simulink library "Single_Track_Model_linear"  (R2018b)
settings: Solver=VariableStepAuto  StartTime=0.0  StopTime=10.0  RelTol=1e-3
undefined symbols (not defined in the file): DiscIntNeverNeededParam, par_TIR, par_VEH, psi0, psip0, v0
libraries: simulink x2, vehicle_model x1
(part 1 of 2)
settings Model: Creator=Johannes  LastModifiedBy=Tony
settings SFSimCC: SimUseLocalCustomCode=off
settings RTWCC: RTWUseLocalCustomCode=off

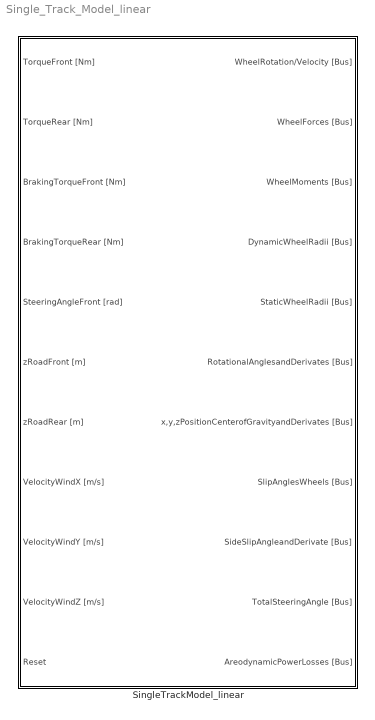
== system Single_Track_Model_linear ==
  SingleTrackModel_linear : Subsystem  mask(SB){RohAir=1.204, VEH_m=2.16e+03, VEH_Iz=5100, VEH_xSP=1.43, VEH_g=9.81, VEH_cz=0, VEH_cx=0.29, VEH_cy=0, VEH_Afront=2.24, VEH_xDP=1.43, VEH_yDP=0, VEH_l=2.968, INIT_x=0, INIT_y=0, INIT_psi=psi0, psip0=psip0, INIT_zroad_RF0=0, INIT_zroad_LF0=0, INIT_zroad_RR0=0, INIT_zroad_LR0=0, v0=v0, unloadedRadius_F=0.339750, c_alpha_F=1.034891575000098e+05, unloadedRadius_R=0.336500, c_alpha_R=1.056481395191441e+05}
      mask prompts: RohAir "Air Density [kg/m^3]"; VEH_m "Mass Vehicle [kg]"; VEH_Iz "Inertia of Vehicle about z [kg m^2]"; VEH_xSP "Center of Gravity of Vehicle in x [m]"; VEH_g "Gravity [N/kg]"; VEH_cz "cw-Value in z [-]"; VEH_cx "cw-Value in x [-]"; VEH_cy "cw-Value in y [-]"; VEH_Afront "Front Surface area [m^2]"; VEH_xDP "Pressure point position in x-direction [m]"; VEH_yDP "Pressure point position in y-direction [m]"; VEH_l "Wheel Base [m]"; INIT_x "Initial Position x"; INIT_y "Initial Position y"; INIT_psi "Initial Position psi"; psip0 "Initial psip"; INIT_zroad_RF0 "Initial Road Position z Right Front"; INIT_zroad_LF0 "Initial Road Position z Left Front"; INIT_zroad_RR0 "Initial Road Position z Right Rear"; INIT_zroad_LR0 "Initial Road Position z Left Rear"; v0 "Initial Speed [m/s]"; unloadedRadius_F "Unloaded Radius Front Tire"; c_alpha_F "Lateral Stiffness Front"; unloadedRadius_R "Unloaded Radius Rear Tire"; c_alpha_R "Lateral Stiffness Rear"
      mask help:
      | <Author> Johannes Rühm
      | <Date> 05/12/2018
      |
      | <Description>
      | Single Track Model using a linear tire model. Structure is based on double track model of "Schultze". Lateral Stiffnesses of tires must be calculated with double track model.
      |
      | <Parameters>
      | ...
      |
      | <Inputs>
      | TorqueFront [Nm]
      | TorqueRear [Nm]
      | BrakingTorqueFront [Nm]
      | BrakingTorqueRear [Nm]
      | SteeringAngleFront [rad]
      | zRoadFront [m]
      | zRoadRear [m]
      | VelocityWindX [m/s]
      | VelocityWindY [m/s]
      | VelocityWindZ [m/s]
      | Reset
      |
      | <Outputs>
      | WheelRotation/Velocity [Bus]
      | WheelForces [Bus]
      | WheelMoments [Bus]
      | DynamicWheelRadii [Bus]
      | StaticWheelRadii [Bus]
      | RotaionalAnglesandDerivatives [Bus]
      | x,y,zPositionCenterofGravityandDerivates [Bus]
      | SlipAnglesWheels [Bus]
      | SideSlipAngleandDerivate [Bus]
      | TotalSteeringAngle [Bus]
      | AreodynamicPowerLosses [Bus]
      mask init:
      | %savedec=0;
      | [par_VEH, par_TIR] =  Init_ESM_linear (RohAir,VEH_m,VEH_xSP,VEH_g,VEH_cz,VEH_cx,VEH_cy,VEH_xDP,VEH_yDP,VEH_Iz,VEH_l,VEH_Afront, unloadedRadius_F, c_alpha_F, unloadedRadius_R, c_alpha_R)
      mask DialogControl Container12 Prompt: Vehicle
      mask DialogControl Container13 Prompt: Mass Data
      mask DialogControl Container15 Prompt: Aerodynamics
      mask DialogControl Container18 Prompt: Dimensions
      mask DialogControl Container32 Prompt: Initial Parameters
      mask DialogControl Container4 Prompt: Tire
      mask DialogControl Container6 Prompt: Front
      mask DialogControl Container8 Prompt: Rear

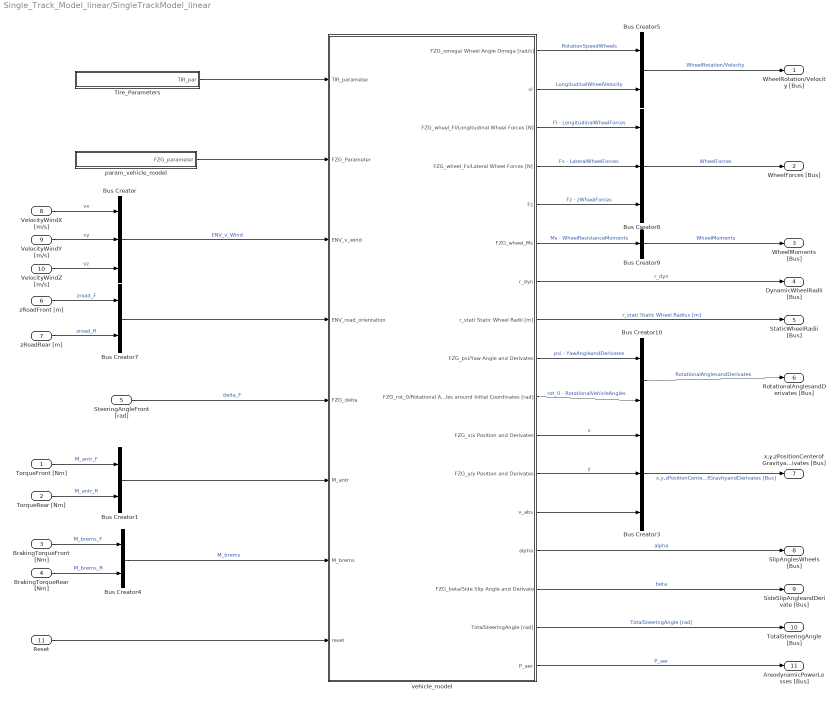
== system Single_Track_Model_linear/SingleTrackModel_linear ==
  TorqueFront [Nm] : Inport
  TorqueRear [Nm] : Inport  Port=2
  BrakingTorqueFront [Nm] : Inport  Port=3
  BrakingTorqueRear [Nm] : Inport  Port=4
  SteeringAngleFront [rad] : Inport  Port=5
  zRoadFront [m] : Inport  Port=6
  zRoadRear [m] : Inport  Port=7
  VelocityWindX [m/s] : Inport  Port=8
  VelocityWindY [m/s] : Inport  Port=9
  VelocityWindZ [m/s] : Inport  Port=10
  Reset : Inport  Port=11
  Bus Creator : BusCreator  Inputs=3
  Bus Creator{1,4..5,7,10} (5 alike) : BusCreator  Inputs=2
  Bus Creator3 : BusCreator  Inputs=3
  Bus Creator8 : BusCreator  Inputs=3
  Bus Creator9 : BusCreator  Inputs=1
  Tire_Parameters : Subsystem
  param_vehicle_model : Subsystem
  vehicle_model : Subsystem  TreatAsAtomicUnit=on
      settings: MinAlgLoopOccurrences=on
  WheelRotation/Velocity [Bus] : Outport
  WheelForces [Bus] : Outport  Port=2
  WheelMoments [Bus] : Outport  Port=3
  DynamicWheelRadii [Bus] : Outport  Port=4
  StaticWheelRadii [Bus] : Outport  Port=5
  RotationalAnglesandDerivates [Bus] : Outport  Port=6
  x,y,zPositionCenterofGravityandDerivates [Bus] : Outport  Port=7
  SlipAnglesWheels [Bus] : Outport  Port=8
  SideSlipAngleandDerivate [Bus] : Outport  Port=9
  TotalSteeringAngle [Bus] : Outport  Port=10
  AreodynamicPowerLosses [Bus] : Outport  Port=11
  wires:
  Bus Creator4/1 -> vehicle_model/7(M_brems)  "M_brems"
  Bus Creator10/1 -> RotationalAnglesandDerivates [Bus]/1  "RotationalAnglesandDerivates"
  Bus Creator9/1 -> WheelMoments [Bus]/1  "WheelMoments"
  Bus Creator8/1 -> WheelForces [Bus]/1  "WheelForces"
  Bus Creator5/1 -> WheelRotation/Velocity [Bus]/1  "WheelRotation/Velocity"
  Bus Creator3/1 -> x,y,zPositionCenterofGravityandDerivates [Bus]/1  "x,y,zPositionCenterofGravityandDerivates [Bus]"
  vehicle_model/10(FZG_rot_0/Rotational Angles around Initial Coordinates [rad]) -> Bus Creator10/2  "rot_0 - RotationalVehicleAngles"
  vehicle_model/6(FZG_wheel_Ms) -> Bus Creator9/1  "Ms - WheelResistanceMoments"
  vehicle_model/4(FZG_wheel_Fs/Lateral Wheel Forces [N]) -> Bus Creator8/2  "Fs - LateralWheelForces"
  vehicle_model/15(FZG_beta/Side Slip Angle and Derivate) -> SideSlipAngleandDerivate [Bus]/1  "beta"
  vehicle_model/3(FZG_wheel_Fl/Longitudinal Wheel Forces [N]) -> Bus Creator8/1  "Fl - LongitudinalWheelForces"
  vehicle_model/12(FZG_y/y Position and Derivates) -> Bus Creator3/2  "y"
  vehicle_model/11(FZG_x/x Position and Derivates) -> Bus Creator3/1  "x"
  vehicle_model/9(FZG_psi/Yaw Angle and Derivates) -> Bus Creator10/1  "psi - YawAngleandDerivates"
  vehicle_model/1(FZG_omega/ Wheel Angle Omega [rad/s]) -> Bus Creator5/1  "RotationSpeedWheels"
  vehicle_model/7(r_dyn) -> DynamicWheelRadii [Bus]/1  "r_dyn"
  param_vehicle_model/1(FZG_parameter) -> vehicle_model/2(FZG_Parameter)
  vehicle_model/2(vl) -> Bus Creator5/2  "LongitudinalWheelVelocity"
  TorqueFront [Nm]/1 -> Bus Creator1/1  "M_antr_F"
  Tire_Parameters/1(TIR_par) -> vehicle_model/1(TIR_parameter)
  VelocityWindZ [m/s]/1 -> Bus Creator/3  "vz"
  VelocityWindY [m/s]/1 -> Bus Creator/2  "vy"
  VelocityWindX [m/s]/1 -> Bus Creator/1  "vx"
  Bus Creator/1 -> vehicle_model/3(ENV_v_wind)  "ENV_v_Wind"
  TorqueRear [Nm]/1 -> Bus Creator1/2  "M_antr_R"
  Bus Creator1/1 -> vehicle_model/6(M_antr)
  BrakingTorqueFront [Nm]/1 -> Bus Creator4/1  "M_brems_F"
  BrakingTorqueRear [Nm]/1 -> Bus Creator4/2  "M_brems_R"
  Reset/1 -> vehicle_model/8(reset)
  SteeringAngleFront [rad]/1 -> vehicle_model/5(FZG_delta)  "delta_F"
  zRoadFront [m]/1 -> Bus Creator7/1  "zroad_F"
  zRoadRear [m]/1 -> Bus Creator7/2  "zroad_R"
  Bus Creator7/1 -> vehicle_model/4(ENV_road_orientation)
  vehicle_model/17(P_aer) -> AreodynamicPowerLosses [Bus]/1  "P_aer"
  vehicle_model/16(TotalSteeringAngle [rad]) -> TotalSteeringAngle [Bus]/1  "TotalSteeringAngle [rad]"
  vehicle_model/14(alpha) -> SlipAnglesWheels [Bus]/1  "alpha"
  vehicle_model/8(r_stat/ Static Wheel Radii [m]) -> StaticWheelRadii [Bus]/1  "r_stat/ Static Wheel Radius [m]"
  vehicle_model/5(Fz) -> Bus Creator8/3  "Fz - zWheelForces"
  vehicle_model/13(v_abs) -> Bus Creator3/3

== system Single_Track_Model_linear/SingleTrackModel_linear/Tire_Parameters ==
  param_tire_model : Subsystem
  TIR_par : Outport
  wires:
  param_tire_model/1(TIR_parameter) -> TIR_par/1

== system Single_Track_Model_linear/SingleTrackModel_linear/param_vehicle_model ==
  Bus Creator : BusCreator  Inputs=13
  Constant : Constant  Value=par_VEH.m
  Constant1 : Constant  Value=par_VEH.cz
  Constant2 : Constant  Value=par_VEH.RohAir
  Constant23 : Constant  Value=par_VEH.lDP
  Constant24 : Constant  Value=par_VEH.lF
  Constant25 : Constant  Value=par_VEH.lR
  Constant28 : Constant  Value=par_VEH.g
  Constant31 : Constant  Value=par_VEH.cx
  Constant32 : Constant  Value=par_VEH.Afront
  Constant34 : Constant  Value=par_VEH.cy
  Constant5 : Constant  Value=par_VEH.Iz
  Constant6 : Constant  Value=par_VEH.xSP
  Constant9 : Constant  Value=par_VEH.l
  FZG_parameter : Outport
  wires:
  Constant1/1 -> Bus Creator/2  "cz"
  Constant23/1 -> Bus Creator/13  "lDP"
  Constant34/1 -> Bus Creator/12  "cy"
  Constant2/1 -> Bus Creator/11  "rhoair"
  Constant32/1 -> Bus Creator/10  "Afront"
  Constant31/1 -> Bus Creator/9  "cx"
  Bus Creator/1 -> FZG_parameter/1
  Constant/1 -> Bus Creator/1  "m"
  Constant5/1 -> Bus Creator/3  "Iz"
  Constant6/1 -> Bus Creator/4  "xSP"
  Constant9/1 -> Bus Creator/5  "l"
  Constant24/1 -> Bus Creator/6  "lF"
  Constant25/1 -> Bus Creator/7  "lR"
  Constant28/1 -> Bus Creator/8  "g"

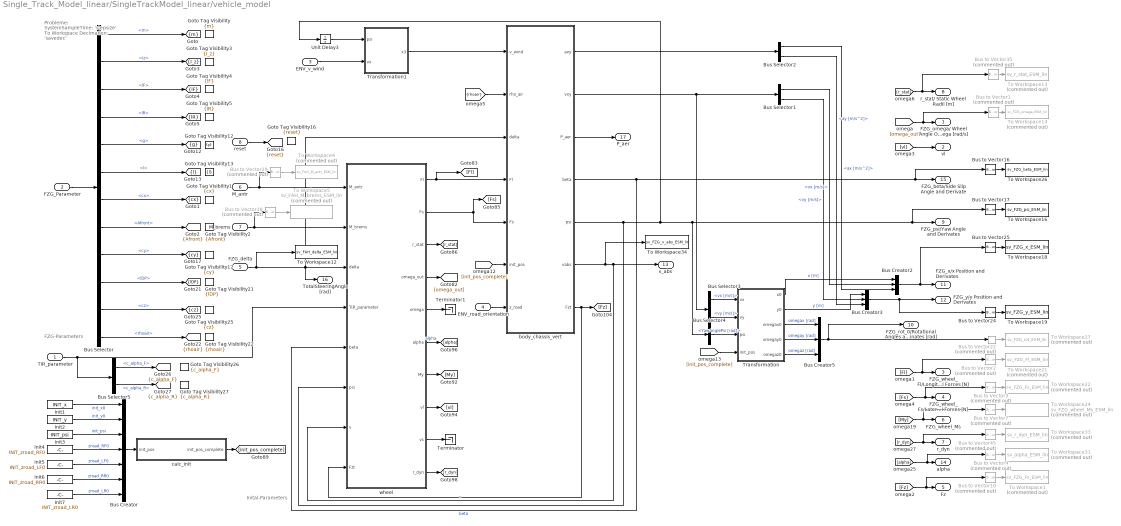
== system Single_Track_Model_linear/SingleTrackModel_linear/vehicle_model ==
  note: Probleme:
      | SystemSampleTime: 'stepsize'
      |
      |
      | To Workspace
      | Decimation: 'savedec'
  note: FZG-Parameters
  note: Inital-Parameters
  TIR_parameter : Inport
  FZG_Parameter : Inport  Port=2
  ENV_v_wind : Inport  Port=3
  ENV_road_orientation : Inport  Port=4
  FZG_delta : Inport  Port=5
  M_antr : Inport  Port=6  PortDimensions=2
  M_brems : Inport  Port=7  PortDimensions=2
  reset : Inport  Port=8
  Bus Creator : BusCreator  Inputs=7
  Bus Creator2 : BusCreator  Inputs=3
  Bus Creator3 : BusCreator  Inputs=3
  Bus Creator5 : BusCreator  Inputs=3
  Bus Selector : BusSelector  OutputSignals=m,Iz,lF,lR,g,l,cx,Afront,cy,lDP,cz,rhoair
  Bus Selector1 : BusSelector  OutputSignals=vx [m/s],vy [m/s]
  Bus Selector2 : BusSelector  OutputSignals=ax [m/s^2],ay [m/s^2]
  Bus Selector3 : BusSelector  OutputSignals=vx [m/s],vy [m/s]
  Bus Selector4 : BusSelector  OutputSignals=YawAnglePsi [rad]
  Bus Selector5 : BusSelector  OutputSignals=front.c_alpha_F,rear.c_alpha_R
  Bus to Vector{1..4,7,10,22,29,35,38,45} (11 alike) : BusToVector  Commented=on
  Bus to Vector{16..17,24..25} (4 alike) : BusToVector
  Goto Tag Visibility : GotoTagVisibility  GotoTag=m
  Goto Tag Visibility1 : GotoTagVisibility  GotoTag=cx
  Goto Tag Visibility12 : GotoTagVisibility  GotoTag=g
  Goto Tag Visibility13 : GotoTagVisibility  GotoTag=l
  Goto Tag Visibility16 : GotoTagVisibility  GotoTag=reset
  Goto Tag Visibility17 : GotoTagVisibility  GotoTag=cy
  Goto Tag Visibility2 : GotoTagVisibility  GotoTag=Afront
  Goto Tag Visibility21 : GotoTagVisibility  GotoTag=lDP
  Goto Tag Visibility22 : GotoTagVisibility  GotoTag=rhoair
  Goto Tag Visibility25 : GotoTagVisibility  GotoTag=cz
  Goto Tag Visibility26 : GotoTagVisibility  GotoTag=c_alpha_F
  Goto Tag Visibility27 : GotoTagVisibility  GotoTag=c_alpha_R
  Goto Tag Visibility3 : GotoTagVisibility  GotoTag=I_z
  Goto Tag Visibility4 : GotoTagVisibility  GotoTag=lF
  Goto Tag Visibility5 : GotoTagVisibility  GotoTag=lR
  Init1 : Constant  Value=INIT_x
  Init2 : Constant  Value=INIT_y
  Init3 : Constant  Value=INIT_psi
  Init4 : Constant  Value=INIT_zroad_RF0
  Init5 : Constant  Value=INIT_zroad_LF0
  Init6 : Constant  Value=INIT_zroad_RR0
  Init7 : Constant  Value=INIT_zroad_LR0
  Terminator : Terminator
  Terminator1 : Terminator
  To Workspace1 : ToWorkspace  Commented=on  VariableName=sv_FZG_Fz_ESM_lin  SampleTime=-1
      settings: Decimation=savedec  Save2DSignal=2-D array (concatenate along first dimension)
  To Workspace12 : ToWorkspace  VariableName=sv_FAH_delta_ESM_lin  SampleTime=-1
      settings: Decimation=savedec  Save2DSignal=2-D array (concatenate along first dimension)
  To Workspace13 : ToWorkspace  Commented=on  VariableName=sv_r_stat_ESM_lin  SampleTime=-1
      settings: Decimation=savedec  Save2DSignal=2-D array (concatenate along first dimension)
  To Workspace14 : ToWorkspace  Commented=on  VariableName=sv_FZG_omega_ESM_lin  SampleTime=-1
      settings: Decimation=savedec  Save2DSignal=2-D array (concatenate along first dimension)
  To Workspace16 : ToWorkspace  VariableName=sv_FZG_psi_ESM_lin  SampleTime=-1
      settings: Decimation=savedec  Save2DSignal=2-D array (concatenate along first dimension)
  To Workspace18 : ToWorkspace  VariableName=sv_FZG_x_ESM_lin  SampleTime=-1
      settings: Decimation=savedec  Save2DSignal=2-D array (concatenate along first dimension)
  To Workspace19 : ToWorkspace  VariableName=sv_FZG_y_ESM_lin  SampleTime=-1
      settings: Decimation=savedec  Save2DSignal=2-D array (concatenate along first dimension)
  To Workspace21 : ToWorkspace  Commented=on  VariableName=sv_FZG_Fl_ESM_lin  SampleTime=-1
      settings: Decimation=savedec  Save2DSignal=2-D array (concatenate along first dimension)
  To Workspace22 : ToWorkspace  Commented=on  VariableName=sv_FZG_Fs_ESM_lin  SampleTime=-1
      settings: Decimation=savedec  Save2DSignal=2-D array (concatenate along first dimension)
  To Workspace24 : ToWorkspace  Commented=on  VariableName=sv_FZG_wheel_Ms_ESM_lin  SampleTime=-1
      settings: Decimation=savedec  Save2DSignal=2-D array (concatenate along first dimension)
  To Workspace26 : ToWorkspace  VariableName=sv_FZG_beta_ESM_lin  SampleTime=-1
      settings: Decimation=savedec  Save2DSignal=2-D array (concatenate along first dimension)
  To Workspace27 : ToWorkspace  Commented=on  VariableName=sv_FZG_rot_ESM_lin  SampleTime=-1
      settings: Decimation=savedec  Save2DSignal=2-D array (concatenate along first dimension)
  To Workspace31 : ToWorkspace  Commented=on  VariableName=sv_alpha_ESM_lin  SampleTime=-1
      settings: Decimation=savedec  Save2DSignal=2-D array (concatenate along first dimension)
  To Workspace33 : ToWorkspace  Commented=on  VariableName=sv_r_dyn_ESM_lin  SampleTime=-1
      settings: Decimation=savedec  Save2DSignal=2-D array (concatenate along first dimension)
  To Workspace34 : ToWorkspace  VariableName=sv_FZG_v_abs_ESM_lin  SampleTime=-1
      settings: Decimation=savedec  Save2DSignal=2-D array (concatenate along first dimension)
  To Workspace4 : ToWorkspace  Commented=on  VariableName=sv_FAH_M_antr_ESM_lin  SampleTime=-1
      settings: Decimation=savedec  Save2DSignal=2-D array (concatenate along first dimension)
  To Workspace5 : ToWorkspace  Commented=on  VariableName=sv_FAH_M_brems_ESM_lin  SampleTime=-1
      settings: Decimation=savedec  Save2DSignal=2-D array (concatenate along first dimension)
  Transformation : Subsystem
  Transformation1 : Subsystem
  Unit Delay3 : UnitDelay  SampleTime=-1
  body_chassis_vert : Subsystem
  calc_init : Subsystem
  wheel : Subsystem
  FZG_omega/ Wheel Angle Omega [rad/s] : Outport
  vl : Outport  Port=2
  FZG_wheel_Fl/Longitudinal Wheel Forces [N] : Outport  Port=3
  FZG_wheel_Fs/Lateral Wheel Forces [N] : Outport  Port=4
  Fz : Outport  Port=5
  FZG_wheel_Ms : Outport  Port=6
  r_dyn : Outport  Port=7
  r_stat/ Static Wheel Radii [m] : Outport  Port=8
  FZG_psi/Yaw Angle and Derivates : Outport  Port=9
  FZG_rot_0/Rotational Angles around Initial Coordinates [rad] : Outport  Port=10
  FZG_x/x Position and Derivates : Outport  Port=11  PortDimensions=3
  FZG_y/y Position and Derivates : Outport  Port=12
  v_abs : Outport  Port=13
  alpha : Outport  Port=14
  FZG_beta/Side Slip Angle and Derivate : Outport  Port=15
  TotalSteeringAngle [rad] : Outport  Port=16
  P_aer : Outport  Port=17
  tag scope: Afront=scoped, I_z=scoped, c_alpha_F=scoped, c_alpha_R=scoped, cx=scoped, cy=scoped, cz=scoped, g=scoped, l=scoped, lDP=scoped, lF=scoped, lR=scoped, m=scoped, reset=scoped, rhoair=scoped
  wires:
  M_antr/1 -> wheel/1(M_antr), Bus to Vector29/1
  Bus to Vector29/1 -> To Workspace4/1
  M_brems/1 -> wheel/2(M_brems), Bus to Vector38/1
  Bus to Vector38/1 -> To Workspace5/1
  FZG_delta/1 -> TotalSteeringAngle [rad]/1, wheel/3(delta), body_chassis_vert/3(delta), To Workspace12/1
  Bus to Vector2/1 -> To Workspace21/1
  Bus to Vector25/1 -> To Workspace18/1
  Bus Creator5/1 -> Bus to Vector22/1, FZG_rot_0/Rotational Angles around Initial Coordinates [rad]/1
  Bus to Vector4/1 -> To Workspace31/1
  Bus to Vector1/1 -> To Workspace14/1
  Bus to Vector16/1 -> To Workspace26/1
  Bus to Vector24/1 -> To Workspace19/1
  [omega_out] -> FZG_omega/ Wheel Angle Omega [rad/s]/1, Bus to Vector1/1
  Bus to Vector17/1 -> To Workspace16/1
  Bus Creator3/1 -> Bus to Vector24/1, FZG_y/y Position and Derivates/1
  Bus to Vector3/1 -> To Workspace22/1
  Bus to Vector7/1 -> To Workspace24/1
  Bus to Vector35/1 -> To Workspace13/1
  Bus to Vector45/1 -> To Workspace33/1
  [Fl] -> FZG_wheel_Fl/Longitudinal Wheel Forces [N]/1, Bus to Vector2/1
  body_chassis_vert/5(psi) -> wheel/6(psi), Unit Delay3/1, Bus Selector4/1, FZG_psi/Yaw Angle and Derivates/1, Bus to Vector17/1
  [Fs] -> FZG_wheel_Fs/Lateral Wheel Forces [N]/1, Bus to Vector3/1
  [r_dyn] -> r_dyn/1, Bus to Vector45/1
  [My] -> FZG_wheel_Ms/1, Bus to Vector7/1
  Bus to Vector10/1 -> To Workspace1/1
  body_chassis_vert/4(beta) -> wheel/5(beta), FZG_beta/Side Slip Angle and Derivate/1, Bus to Vector16/1  "beta"
  [Fz] -> Fz/1, Bus to Vector10/1
  Bus Creator2/1 -> FZG_x/x Position and Derivates/1, Bus to Vector25/1
  [r_stat] -> r_stat/ Static Wheel Radii [m]/1, Bus to Vector35/1
  [alpha] -> alpha/1, Bus to Vector4/1
  Bus to Vector22/1 -> To Workspace27/1
  Bus Selector5/2 -> [c_alpha_R]  "<c_alpha_R>"
  Bus Selector5/1 -> [c_alpha_F]  "<c_alpha_F>"
  Init7/1 -> Bus Creator/7  "zroad_LR0"
  Init6/1 -> Bus Creator/6  "zroad_RR0"
  Init5/1 -> Bus Creator/5  "zroad_LF0"
  Init4/1 -> Bus Creator/4  "zroad_RF0"
  Init3/1 -> Bus Creator/3  "init_psi"
  Init2/1 -> Bus Creator/2  "init_y0"
  Init1/1 -> Bus Creator/1  "init_x0"
  [vl] -> vl/1
  wheel/10(r_dyn) -> [r_dyn]
  wheel/6(alpha) -> [alpha]  "alpha"
  wheel/9(vs) -> Terminator/1
  wheel/8(vl) -> [vl]
  wheel/7(My) -> [My]
  wheel/3(r_stat) -> [r_stat]
  [init_pos_complete] -> Transformation/4(init_pos)
  [init_pos_complete] -> body_chassis_vert/6(init_pos)
  calc_init/1(init_pos_complete) -> [init_pos_complete]
  TIR_parameter/1 -> Bus Selector5/1, wheel/4(TIR_parameter)
  wheel/5(omega) -> Terminator1/1
  wheel/4(omega_out) -> [omega_out]
  body_chassis_vert/3(P_aer) -> P_aer/1
  Bus Selector/7 -> [cx]  "<cx>"
  Bus Selector/8 -> [Afront]  "<Afront>"
  Bus Selector/10 -> [lDP]  "<lDP>"
  Bus Selector/11 -> [cz]  "<cz>"
  body_chassis_vert/1(axy) -> Bus Selector2/1
  body_chassis_vert/2(vxy) -> Bus Selector1/1, Bus Selector3/1
  Bus Selector/9 -> [cy]  "<cy>"
  Unit Delay3/1 -> Transformation1/1(psi)
  Transformation1/1(x3) -> body_chassis_vert/1(v_wind)
  Bus Creator/1 -> calc_init/1(init_pos)
  Transformation/5(omegaz0) -> Bus Creator5/3  "omegaz [rad]"
  Transformation/4(omegay0) -> Bus Creator5/2  "omegay [rad]"
  Transformation/3(omegax0) -> Bus Creator5/1  "omegax [rad]"
  Bus Selector4/1 -> Transformation/3(psi)  "<YawAnglePsi [rad]>"
  Bus Selector3/2 -> Transformation/2(vy)  "<vy [m/s]>"
  Bus Selector3/1 -> Transformation/1(vx)  "<vx [m/s]>"
  Transformation/2(y0) -> Bus Creator3/1  "y [m]"
  Transformation/1(x0) -> Bus Creator2/1  "x [m]"
  ENV_road_orientation/1 -> body_chassis_vert/7(z_road)
  [rhoair] -> body_chassis_vert/2(rho_air)
  ENV_v_wind/1 -> Transformation1/2(vx)
  FZG_Parameter/1 -> Bus Selector/1
  wheel/2(Fs) -> body_chassis_vert/5(Fs), [Fs]
  body_chassis_vert/6(vabs) -> wheel/7(v), v_abs/1, To Workspace34/1  "v"
  Bus Selector/1 -> [m]  "<m>"
  Bus Selector/2 -> [I_z]  "<Iz>"
  Bus Selector/3 -> [lF]  "<lF>"
  Bus Selector/4 -> [lR]  "<lR>"
  Bus Selector/5 -> [g]  "<g>"
  Bus Selector/6 -> [l]  "<l>"
  wheel/1(Fl) -> body_chassis_vert/4(Fl), [Fl]
  Bus Selector1/1 -> Bus Creator2/2  "<vx [m/s]>"
  Bus Selector1/2 -> Bus Creator3/2  "<vy [m/s]>"
  Bus Selector2/1 -> Bus Creator2/3  "<ax [m/s^2]>"
  Bus Selector2/2 -> Bus Creator3/3  "<ay [m/s^2]>"
  reset/1 -> [reset]
  body_chassis_vert/7(Fzt) -> [Fz], wheel/8(Fzt)
  Bus Selector/12 -> [rhoair]  "<rhoair>"

== system Single_Track_Model_linear/SingleTrackModel_linear/Tire_Parameters/param_tire_model ==
  note: TIRE DATA
  note: TIRE DATA
  Bus Creator : BusCreator  Inputs=2
  Bus Creator2 : BusCreator  Inputs=2
  Bus Creator4 : BusCreator  Inputs=2
  Constant : Constant  Value=par_TIR(2).unloadedRadius
  Constant1 : Constant  Value=par_TIR(1).c_alpha_F
  Constant137 : Constant  Value=par_TIR(1).unloadedRadius
  Constant2 : Constant  Value=par_TIR(2).c_alpha_R
  TIR_parameter : Outport
  wires:
  Constant2/1 -> Bus Creator/2  "c_alpha_R"
  Constant1/1 -> Bus Creator2/2  "c_alpha_F"
  Constant137/1 -> Bus Creator2/1  "UNLOADED_RADIUS"
  Constant/1 -> Bus Creator/1  "UNLOADED_RADIUS"
  Bus Creator/1 -> Bus Creator4/2  "rear"
  Bus Creator2/1 -> Bus Creator4/1  "front"
  Bus Creator4/1 -> TIR_parameter/1

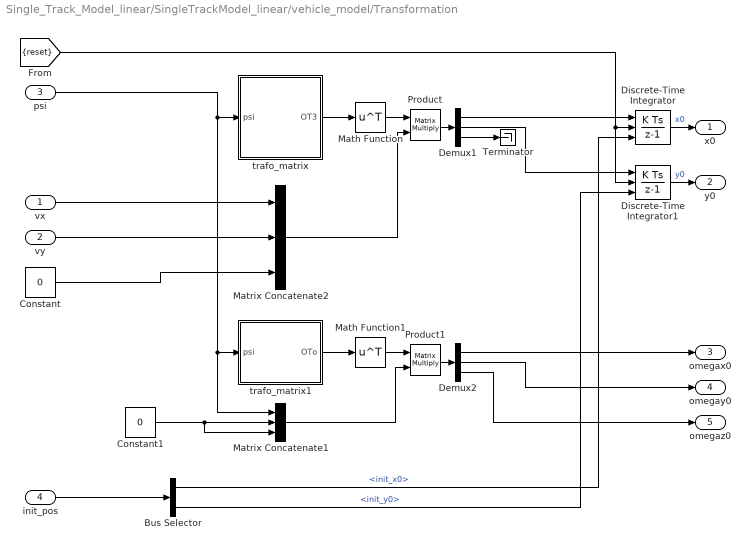
== system Single_Track_Model_linear/SingleTrackModel_linear/vehicle_model/Transformation ==
  vx : Inport
  vy : Inport  Port=2
  psi : Inport  Port=3
  init_pos : Inport  Port=4
  Bus Selector : BusSelector  OutputSignals=init_x0,init_y0
  Constant : Constant  Value=0
  Constant1 : Constant  Value=0
  Demux1 : Demux  Outputs=3
  Demux2 : Demux  Outputs=3
  Discrete-Time Integrator : DiscreteIntegrator  ExternalReset=sampled level  InitialConditionSource=external  SampleTime=-1  ICPrevOutput=DiscIntNeverNeededParam  ICPrevScaledInput=DiscIntNeverNeededParam
  Discrete-Time Integrator1 : DiscreteIntegrator  ExternalReset=sampled level  InitialConditionSource=external  SampleTime=-1  ICPrevOutput=DiscIntNeverNeededParam  ICPrevScaledInput=DiscIntNeverNeededParam
  Math Function : Math  Operator=transpose  SaturateOnIntegerOverflow=on
  Math Function1 : Math  Operator=transpose  SaturateOnIntegerOverflow=on
  Matrix Concatenate1 : Concatenate  NumInputs=3
  Matrix Concatenate2 : Concatenate  NumInputs=3
  Product : Product  Multiplication=Matrix(*)
  Product1 : Product  Multiplication=Matrix(*)
  Terminator : Terminator
  trafo_matrix : Subsystem
  trafo_matrix1 : Subsystem
  x0 : Outport
  y0 : Outport  Port=2
  omegax0 : Outport  Port=3
  omegay0 : Outport  Port=4
  omegaz0 : Outport  Port=5
  wires:
  Product1/1 -> Demux2/1
  trafo_matrix1/1(OTo) -> Math Function1/1
  Math Function1/1 -> Product1/1
  Matrix Concatenate1/1 -> Product1/2
  Product/1 -> Demux1/1
  Demux1/3 -> Terminator/1
  Math Function/1 -> Product/1
  Constant/1 -> Matrix Concatenate2/3
  Matrix Concatenate2/1 -> Product/2
  trafo_matrix/1(OT3) -> Math Function/1
  Bus Selector/2 -> Discrete-Time Integrator1/3  "<init_y0>"
  Bus Selector/1 -> Discrete-Time Integrator/3  "<init_x0>"
  init_pos/1 -> Bus Selector/1
  Demux2/3 -> omegaz0/1
  Demux2/2 -> omegay0/1
  Demux2/1 -> omegax0/1
  Discrete-Time Integrator1/1 -> y0/1  "y0"
  Discrete-Time Integrator/1 -> x0/1  "x0"
  vy/1 -> Matrix Concatenate2/2
  vx/1 -> Matrix Concatenate2/1
  psi/1 -> trafo_matrix1/1(psi), Matrix Concatenate1/1, trafo_matrix/1(psi)
  Demux1/2 -> Discrete-Time Integrator1/1
  Demux1/1 -> Discrete-Time Integrator/1
  [reset] -> Discrete-Time Integrator/2, Discrete-Time Integrator1/2
  Constant1/1 -> Matrix Concatenate1/3, Matrix Concatenate1/2

== system Single_Track_Model_linear/SingleTrackModel_linear/vehicle_model/Transformation1 ==
  psi : Inport
  vx : Inport  Port=2
  Bus Creator : BusCreator  Inputs=3
  Bus Selector : BusSelector  OutputSignals=vx,vy,vz
  Bus Selector1 : BusSelector  OutputSignals=YawAnglePsi [rad]
  Demux1 : Demux  Outputs=3
  Math Function : Math  Operator=transpose  SaturateOnIntegerOverflow=on
  Matrix Concatenate2 : Concatenate  NumInputs=3
  Product : Product  Multiplication=Matrix(*)
  trafo_matrix : Subsystem
  x3 : Outport
  wires:
  Product/1 -> Demux1/1
  Math Function/1 -> Product/1
  Matrix Concatenate2/1 -> Product/2
  trafo_matrix/1(OT3) -> Math Function/1
  psi/1 -> Bus Selector1/1
  Demux1/3 -> Bus Creator/3  "vwindz"
  Demux1/2 -> Bus Creator/2  "vwindy"
  Demux1/1 -> Bus Creator/1  "vwindx"
  Bus Selector/3 -> Matrix Concatenate2/3  "<vz>"
  Bus Selector/2 -> Matrix Concatenate2/2  "<vy>"
  Bus Selector/1 -> Matrix Concatenate2/1  "<vx>"
  vx/1 -> Bus Selector/1
  Bus Creator/1 -> x3/1
  Bus Selector1/1 -> trafo_matrix/1(psi)  "<YawAnglePsi [rad]>"

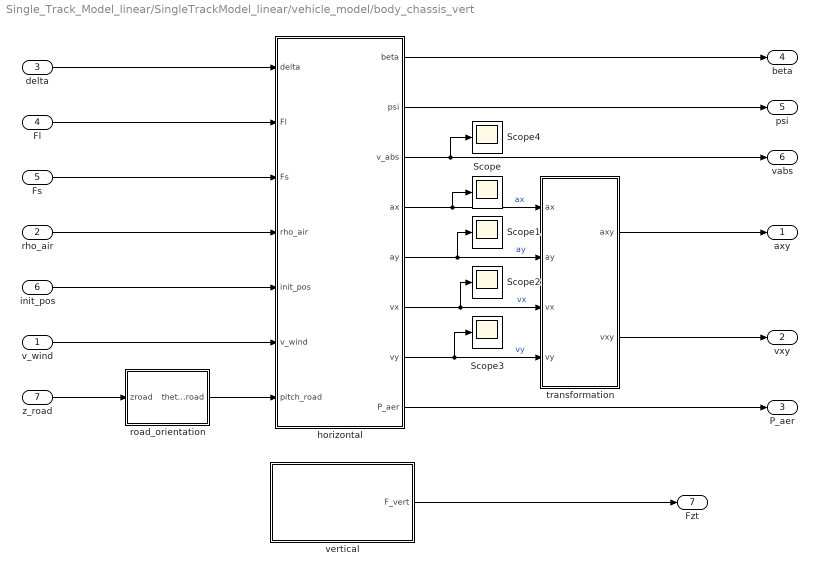
== system Single_Track_Model_linear/SingleTrackModel_linear/vehicle_model/body_chassis_vert ==
  v_wind : Inport
  rho_air : Inport  Port=2
  delta : Inport  Port=3
  Fl : Inport  Port=4
  Fs : Inport  Port=5
  init_pos : Inport  Port=6
  z_road : Inport  Port=7
  Scope{,1..4} (5 alike) : Scope
  horizontal : Subsystem
  road_orientation : Subsystem
  transformation : Subsystem
  vertical : Subsystem
  axy : Outport
  vxy : Outport  Port=2
  P_aer : Outport  Port=3
  beta : Outport  Port=4
  psi : Outport  Port=5
  vabs : Outport  Port=6
  Fzt : Outport  Port=7
  wires:
  road_orientation/1(theta_road) -> horizontal/7(pitch_road)
  z_road/1 -> road_orientation/1(zroad)
  horizontal/6(vx) -> transformation/3(vx), Scope2/1  "vx"
  horizontal/7(vy) -> transformation/4(vy), Scope3/1  "vy"
  horizontal/5(ay) -> transformation/2(ay), Scope1/1  "ay"
  horizontal/4(ax) -> transformation/1(ax), Scope/1  "ax"
  transformation/1(axy) -> axy/1
  transformation/2(vxy) -> vxy/1
  v_wind/1 -> horizontal/6(v_wind)
  init_pos/1 -> horizontal/5(init_pos)
  rho_air/1 -> horizontal/4(rho_air)
  delta/1 -> horizontal/1(delta)
  horizontal/1(beta) -> beta/1
  horizontal/2(psi) -> psi/1
  Fl/1 -> horizontal/2(Fl)
  horizontal/3(v_abs) -> vabs/1, Scope4/1
  Fs/1 -> horizontal/3(Fs)
  horizontal/8(P_aer) -> P_aer/1
  vertical/1(F_vert) -> Fzt/1

== system Single_Track_Model_linear/SingleTrackModel_linear/vehicle_model/calc_init ==
  init_pos : Inport
  Bus Creator : BusCreator  Inputs=9
  Bus Selector : BusSelector  OutputSignals=init_x0,init_y0,init_psi,zroad_RF0,zroad_LF0,zroad_RR0,zroad_LR0
  pitch : Subsystem
  vertical : Subsystem
  init_pos_complete : Outport
  wires:
  Bus Creator/1 -> init_pos_complete/1
  vertical/1(init_z0) -> Bus Creator/9  "init_z0"
  Bus Selector/7 -> Bus Creator/7  "<zroad_LR0>"
  Bus Selector/6 -> Bus Creator/6  "<zroad_RR0>"
  Bus Selector/5 -> Bus Creator/5  "<zroad_LF0>"
  Bus Selector/4 -> Bus Creator/4  "<zroad_RF0>"
  Bus Selector/3 -> Bus Creator/3  "<init_psi>"
  Bus Selector/2 -> Bus Creator/2  "<init_y0>"
  Bus Selector/1 -> Bus Creator/1  "<init_x0>"
  pitch/1(init_theta) -> vertical/2(theta), Bus Creator/8  "init_theta"
  init_pos/1 -> Bus Selector/1, vertical/1(init_pos), pitch/1(init_pos)

== system Single_Track_Model_linear/SingleTrackModel_linear/vehicle_model/wheel ==
  M_antr : Inport
  M_brems : Inport  Port=2
  delta : Inport  Port=3
  TIR_parameter : Inport  Port=4
  beta : Inport  Port=5
  psi : Inport  Port=6
  v : Inport  Port=7
  Fzt : Inport  Port=8
  Tire Model : Subsystem
  calc_omega : Subsystem
  calc_v : Subsystem
  v0_korr : Subsystem
  Fl : Outport
  Fs : Outport  Port=2
  r_stat : Outport  Port=3
  omega_out : Outport  Port=4
  omega : Outport  Port=5
  alpha : Outport  Port=6
  My : Outport  Port=7
  vl : Outport  Port=8
  vs : Outport  Port=9
  r_dyn : Outport  Port=10
  wires:
  M_brems/1 -> Tire Model/2(M_brems)
  Tire Model/1(r_dyn) -> v0_korr/3(r_dyn), calc_omega/2(r_dyn), r_dyn/1
  Tire Model/6(r_stat) -> r_stat/1
  v0_korr/1(omega_out) -> omega_out/1
  Tire Model/2(Fl) -> Fl/1
  Tire Model/4(My) -> My/1
  calc_omega/1(omega) -> omega/1, v0_korr/2(omega)
  calc_v/1(vl) -> calc_omega/1(vl), vl/1, v0_korr/1(vl)
  calc_v/2(vs) -> vs/1
  delta/1 -> calc_v/1(delta), Tire Model/4(delta)
  psi/1 -> calc_v/3(psi), Tire Model/6(psip)
  beta/1 -> calc_v/2(beta), Tire Model/5(beta)
  M_antr/1 -> Tire Model/3(M_antr)
  Tire Model/3(Fs) -> Fs/1
  TIR_parameter/1 -> Tire Model/8(TIR_parameter)
  Tire Model/5(alpha) -> alpha/1
  v/1 -> calc_v/4(v), Tire Model/7(vabs)
  Fzt/1 -> Tire Model/1(Fz)

== system Single_Track_Model_linear/SingleTrackModel_linear/vehicle_model/Transformation/trafo_matrix ==
  psi : Inport
  Constant{,2..4} (4 alike) : Constant  Value=0
  Constant1 : Constant
  Matrix Concatenate : Concatenate  NumInputs=3  Mode=Multidimensional array  ConcatenateDimension=2
  Matrix Concatenate1 : Concatenate  NumInputs=3
  Matrix Concatenate2 : Concatenate  NumInputs=3
  Matrix Concatenate3 : Concatenate  NumInputs=3
  Trigonometric Function : Trigonometry  Operator=cos
  Trigonometric Function7 : Trigonometry
  Unary Minus : UnaryMinus
  OT3 : Outport
  wires:
  Matrix Concatenate/1 -> OT3/1
  Trigonometric Function7/1 -> Unary Minus/1, Matrix Concatenate2/1
  Unary Minus/1 -> Matrix Concatenate1/2
  psi/1 -> Trigonometric Function/1, Trigonometric Function7/1
  Trigonometric Function/1 -> Matrix Concatenate1/1, Matrix Concatenate2/2
  Matrix Concatenate3/1 -> Matrix Concatenate/3
  Matrix Concatenate2/1 -> Matrix Concatenate/2
  Matrix Concatenate1/1 -> Matrix Concatenate/1
  Constant/1 -> Matrix Concatenate3/1
  Constant1/1 -> Matrix Concatenate3/3
  Constant2/1 -> Matrix Concatenate1/3
  Constant3/1 -> Matrix Concatenate2/3
  Constant4/1 -> Matrix Concatenate3/2

== system Single_Track_Model_linear/SingleTrackModel_linear/vehicle_model/Transformation/trafo_matrix1 ==
  psi : Inport
  Constant{,1,3..4} (4 alike) : Constant  Value=0
  Constant2 : Constant
  Matrix Concatenate : Concatenate  NumInputs=3  Mode=Multidimensional array  ConcatenateDimension=2
  Matrix Concatenate1 : Concatenate  NumInputs=3
  Matrix Concatenate2 : Concatenate  NumInputs=3
  Matrix Concatenate3 : Concatenate  NumInputs=3
  Trigonometric Function : Trigonometry  Operator=cos
  Trigonometric Function7 : Trigonometry
  Unary Minus : UnaryMinus
  OTo : Outport
  wires:
  Constant3/1 -> Matrix Concatenate3/2
  Constant2/1 -> Matrix Concatenate3/1
  Constant1/1 -> Matrix Concatenate2/1
  Constant/1 -> Matrix Concatenate1/1
  Matrix Concatenate1/1 -> Matrix Concatenate/1
  Matrix Concatenate2/1 -> Matrix Concatenate/2
  Matrix Concatenate3/1 -> Matrix Concatenate/3
  Trigonometric Function7/1 -> Matrix Concatenate2/3, Unary Minus/1
  psi/1 -> Trigonometric Function7/1, Trigonometric Function/1
  Unary Minus/1 -> Matrix Concatenate1/2
  Trigonometric Function/1 -> Matrix Concatenate1/3, Matrix Concatenate2/2
  Matrix Concatenate/1 -> OTo/1
  Constant4/1 -> Matrix Concatenate3/3

== system Single_Track_Model_linear/SingleTrackModel_linear/vehicle_model/Transformation1/trafo_matrix ==
  psi : Inport
  Constant{,2..4} (4 alike) : Constant  Value=0
  Constant1 : Constant
  Matrix Concatenate : Concatenate  NumInputs=3  Mode=Multidimensional array  ConcatenateDimension=2
  Matrix Concatenate1 : Concatenate  NumInputs=3
  Matrix Concatenate2 : Concatenate  NumInputs=3
  Matrix Concatenate3 : Concatenate  NumInputs=3
  Trigonometric Function : Trigonometry  Operator=cos
  Trigonometric Function7 : Trigonometry
  Unary Minus4 : UnaryMinus
  OT3 : Outport
  wires:
  Matrix Concatenate1/1 -> Matrix Concatenate/1
  Matrix Concatenate2/1 -> Matrix Concatenate/2
  Trigonometric Function7/1 -> Unary Minus4/1, Matrix Concatenate1/2
  Trigonometric Function/1 -> Matrix Concatenate2/2, Matrix Concatenate1/1
  Matrix Concatenate3/1 -> Matrix Concatenate/3
  Matrix Concatenate/1 -> OT3/1
  Unary Minus4/1 -> Matrix Concatenate2/1
  psi/1 -> Trigonometric Function/1, Trigonometric Function7/1
  Constant/1 -> Matrix Concatenate1/3
  Constant1/1 -> Matrix Concatenate3/3
  Constant2/1 -> Matrix Concatenate2/3
  Constant3/1 -> Matrix Concatenate3/1
  Constant4/1 -> Matrix Concatenate3/2

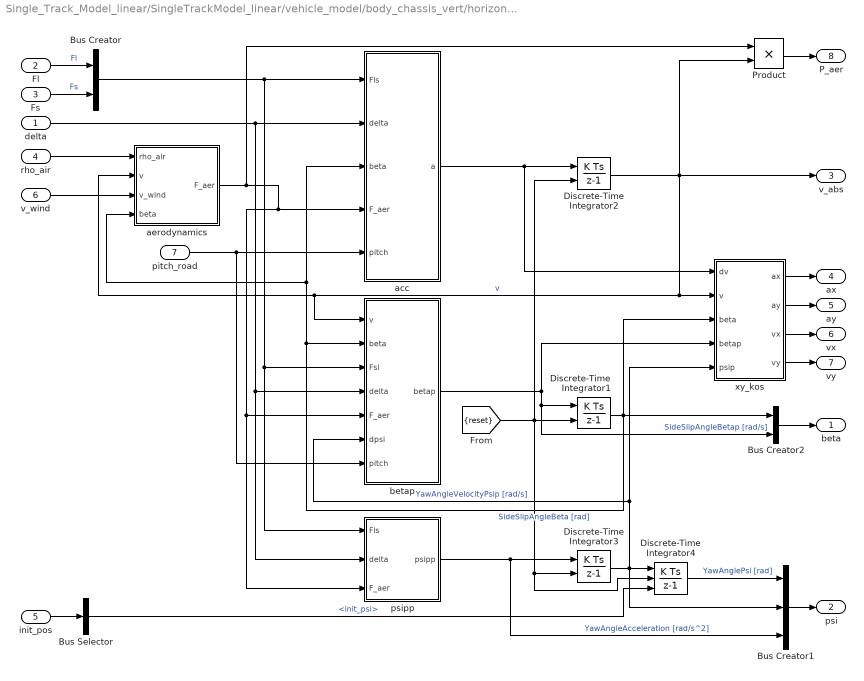
== system Single_Track_Model_linear/SingleTrackModel_linear/vehicle_model/body_chassis_vert/horizontal ==
  delta : Inport
  Fl : Inport  Port=2
  Fs : Inport  Port=3
  rho_air : Inport  Port=4
  init_pos : Inport  Port=5
  v_wind : Inport  Port=6
  pitch_road : Inport  Port=7
  Bus Creator : BusCreator  Inputs=2
  Bus Creator1 : BusCreator  Inputs=3
  Bus Creator2 : BusCreator  Inputs=2
  Bus Selector : BusSelector  OutputSignals=init_psi
  Discrete-Time Integrator1 : DiscreteIntegrator  ExternalReset=sampled level  SampleTime=-1  ICPrevOutput=DiscIntNeverNeededParam  ICPrevScaledInput=DiscIntNeverNeededParam
  Discrete-Time Integrator2 : DiscreteIntegrator  ExternalReset=sampled level  InitialCondition=v0  SampleTime=-1  LimitOutput=on  ICPrevOutput=DiscIntNeverNeededParam  ICPrevScaledInput=DiscIntNeverNeededParam
  Discrete-Time Integrator3 : DiscreteIntegrator  ExternalReset=sampled level  InitialCondition=psip0  SampleTime=-1  ICPrevOutput=DiscIntNeverNeededParam  ICPrevScaledInput=DiscIntNeverNeededParam
  Discrete-Time Integrator4 : DiscreteIntegrator  ExternalReset=sampled level  InitialConditionSource=external  SampleTime=-1  ICPrevOutput=DiscIntNeverNeededParam  ICPrevScaledInput=DiscIntNeverNeededParam
  Product : Product
  acc : Subsystem
  aerodynamics : Subsystem
  betap : Subsystem
  psipp : Subsystem
  xy_kos : Subsystem
  beta : Outport
  psi : Outport  Port=2
  v_abs : Outport  Port=3
  ax : Outport  Port=4
  ay : Outport  Port=5
  vx : Outport  Port=6
  vy : Outport  Port=7
  P_aer : Outport  Port=8
  wires:
  Discrete-Time Integrator2/1 -> v_abs/1, xy_kos/2(v), aerodynamics/2(v), betap/1(v), Product/2  "v"
  Discrete-Time Integrator1/1 -> Bus Creator2/1, aerodynamics/4(beta), acc/3(beta), betap/2(beta), xy_kos/3(beta)  "SideSlipAngleBeta [rad]"
  Bus Creator2/1 -> beta/1
  pitch_road/1 -> betap/7(pitch), acc/5(pitch)
  xy_kos/4(vy) -> vy/1
  xy_kos/2(ay) -> ay/1
  v_wind/1 -> aerodynamics/3(v_wind)
  Bus Selector/1 -> Discrete-Time Integrator4/3  "<init_psi>"
  init_pos/1 -> Bus Selector/1
  [reset] -> Discrete-Time Integrator4/2, Discrete-Time Integrator3/2, Discrete-Time Integrator1/2, Discrete-Time Integrator2/2
  rho_air/1 -> aerodynamics/1(rho_air)
  xy_kos/1(ax) -> ax/1
  Fl/1 -> Bus Creator/1  "Fl"
  Fs/1 -> Bus Creator/2  "Fs"
  Discrete-Time Integrator3/1 -> Discrete-Time Integrator4/1, Bus Creator1/2, xy_kos/5(psip), betap/6(dpsi)  "YawAngleVelocityPsip [rad/s]"
  psipp/1(psipp) -> Discrete-Time Integrator3/1, Bus Creator1/3  "YawAngleAcceleration [rad/s^2]"
  betap/1(betap) -> Bus Creator2/2, Discrete-Time Integrator1/1, xy_kos/4(betap)  "SideSlipAngleBetap [rad/s]"
  delta/1 -> acc/2(delta), psipp/2(delta), betap/4(delta)
  aerodynamics/1(F_aer) -> Product/1, psipp/3(F_aer), betap/5(F_aer), acc/4(F_aer)
  acc/1(a) -> xy_kos/1(dv), Discrete-Time Integrator2/1
  Discrete-Time Integrator4/1 -> Bus Creator1/1  "YawAnglePsi [rad]"
  Bus Creator1/1 -> psi/1
  xy_kos/3(vx) -> vx/1
  Bus Creator/1 -> acc/1(Fls), psipp/1(Fls), betap/3(Fsl)
  Product/1 -> P_aer/1

== system Single_Track_Model_linear/SingleTrackModel_linear/vehicle_model/body_chassis_vert/road_orientation ==
  zroad : Inport
  Bus Selector1 : BusSelector  OutputSignals=zroad_F,zroad_R
  Divide8 : Product  Inputs=*/
  Subtract20 : Sum  Inputs=+-
  Trigonometric Function : Trigonometry  Operator=asin
  theta_road : Outport
  wires:
  Divide8/1 -> Trigonometric Function/1
  [l] -> Divide8/2
  Subtract20/1 -> Divide8/1
  Bus Selector1/1 -> Subtract20/1  "<zroad_F>"
  Trigonometric Function/1 -> theta_road/1
  Bus Selector1/2 -> Subtract20/2  "<zroad_R>"
  zroad/1 -> Bus Selector1/1

== system Single_Track_Model_linear/SingleTrackModel_linear/vehicle_model/body_chassis_vert/transformation ==
  ax : Inport
  ay : Inport  Port=2
  vx : Inport  Port=3
  vy : Inport  Port=4
  Bus Creator1 : BusCreator  Inputs=2
  Bus Creator2 : BusCreator  Inputs=2
  axy : Outport
  vxy : Outport  Port=2
  wires:
  Bus Creator2/1 -> vxy/1
  vy/1 -> Bus Creator2/2  "vy [m/s]"
  vx/1 -> Bus Creator2/1  "vx [m/s]"
  Bus Creator1/1 -> axy/1
  ay/1 -> Bus Creator1/2  "ay [m/s^2]"
  ax/1 -> Bus Creator1/1  "ax [m/s^2]"

== system Single_Track_Model_linear/SingleTrackModel_linear/vehicle_model/body_chassis_vert/vertical ==
  note: Momentengleichgewicht um Vorderrad bzw. Hinterrad --> Vertikalkräfte an Rädern
  Bus Creator1 : BusCreator  Inputs=2
  Divide : Product  Inputs=**/
  Product1 : Product  RndMeth=Zero
  Product3 : Product  RndMeth=Zero
  Signal Conversion2 : SignalConversion  OverrideOpt=off
  Signal Conversion3 : SignalConversion  OverrideOpt=off
  F_vert : Outport
  wires:
  [m] -> Divide/1
  [g] -> Divide/2
  [lR] -> Product3/1
  Bus Creator1/1 -> F_vert/1
  Product3/1 -> Signal Conversion2/1
  Signal Conversion2/1 -> Bus Creator1/1  "F_F"
  Product1/1 -> Signal Conversion3/1
  Signal Conversion3/1 -> Bus Creator1/2  "F_R"
  [l] -> Divide/3
  Divide/1 -> Product1/1, Product3/2
  [lF] -> Product1/2

== system Single_Track_Model_linear/SingleTrackModel_linear/vehicle_model/calc_init/pitch ==
  init_pos : Inport
  Add : Sum
  Add1 : Sum
  Add2 : Sum  Inputs=+-
  Bus Selector : BusSelector  OutputSignals=zroad_RF0,zroad_LF0,zroad_RR0,zroad_LR0
  Divide : Product  Inputs=*/
  Gain : Gain  Gain=0.5
  Gain1 : Gain  Gain=0.5
  Trigonometric Function : Trigonometry  Operator=atan
  init_theta : Outport
  wires:
  Bus Selector/3 -> Add1/1  "<zroad_RR0>"
  Bus Selector/2 -> Add/2  "<zroad_LF0>"
  init_pos/1 -> Bus Selector/1
  Bus Selector/1 -> Add/1  "<zroad_RF0>"
  Add/1 -> Gain/1
  Add1/1 -> Gain1/1
  Bus Selector/4 -> Add1/2  "<zroad_LR0>"
  Gain/1 -> Add2/1
  Gain1/1 -> Add2/2
  Add2/1 -> Divide/1
  Divide/1 -> Trigonometric Function/1
  [l] -> Divide/2
  Trigonometric Function/1 -> init_theta/1

== system Single_Track_Model_linear/SingleTrackModel_linear/vehicle_model/calc_init/vertical ==
  init_pos : Inport
  theta : Inport  Port=2
  Add : Sum
  Add1 : Sum
  Bus Selector : BusSelector  OutputSignals=zroad_RF0,zroad_LF0
  Gain : Gain  Gain=0.5
  Product : Product  RndMeth=Zero
  Trigonometric Function : Trigonometry
  init_z0 : Outport
  wires:
  Add1/1 -> init_z0/1
  Product/1 -> Add1/2
  Trigonometric Function/1 -> Product/2
  theta/1 -> Trigonometric Function/1
  [lF] -> Product/1
  Gain/1 -> Add1/1
  Add/1 -> Gain/1
  Bus Selector/2 -> Add/2  "<zroad_LF0>"
  Bus Selector/1 -> Add/1  "<zroad_RF0>"
  init_pos/1 -> Bus Selector/1

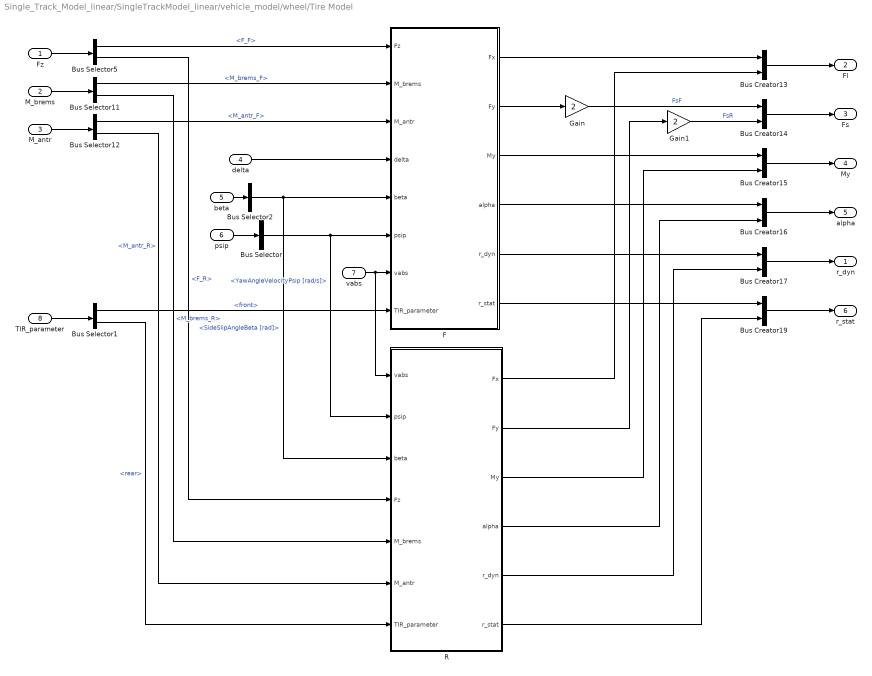
== system Single_Track_Model_linear/SingleTrackModel_linear/vehicle_model/wheel/Tire Model ==
  Fz : Inport
  M_brems : Inport  Port=2
  M_antr : Inport  Port=3
  delta : Inport  Port=4
  beta : Inport  Port=5
  psip : Inport  Port=6
  vabs : Inport  Port=7
  TIR_parameter : Inport  Port=8
  Bus Creator{13..17,19} (6 alike) : BusCreator  Inputs=2
  Bus Selector : BusSelector  OutputSignals=YawAngleVelocityPsip [rad/s]
  Bus Selector1 : BusSelector  OutputSignals=front,rear
  Bus Selector11 : BusSelector  OutputSignals=M_brems_F,M_brems_R
  Bus Selector12 : BusSelector  OutputSignals=M_antr_F,M_antr_R
  Bus Selector2 : BusSelector  OutputSignals=SideSlipAngleBeta [rad]
  Bus Selector5 : BusSelector  OutputSignals=F_F,F_R
  F : Subsystem  mask{mounted_side_input=undefined}
      mask prompts: mounted_side_input "mounted side"
      mask init:
      | switch mounted_side_input
      |     case 1
      |         mounted_side=0;
      |     case 2
      |         mounted_side=1;
      |     case 3
      |         mounted_side=-1;
      | end
      mask TypeOptions mounted_side_input: undefined | left | right
  Gain : Gain  Gain=2
  Gain1 : Gain  Gain=2
  R : Subsystem  mask{mounted_side_input=undefined}
      mask prompts: mounted_side_input "mounted side"
      mask init:
      | switch mounted_side_input
      |     case 1
      |         mounted_side=0;
      |     case 2
      |         mounted_side=1;
      |     case 3
      |         mounted_side=-1;
      | end
      mask TypeOptions mounted_side_input: undefined | left | right
  r_dyn : Outport
  Fl : Outport  Port=2
  Fs : Outport  Port=3
  My : Outport  Port=4
  alpha : Outport  Port=5
  r_stat : Outport  Port=6
  wires:
  Gain1/1 -> Bus Creator14/2  "FsR"
  Gain/1 -> Bus Creator14/1  "FsF"
  beta/1 -> Bus Selector2/1
  psip/1 -> Bus Selector/1
  Fz/1 -> Bus Selector5/1
  Bus Selector5/1 -> F/1(Fz)  "<F_F>"
  Bus Selector5/2 -> R/4(Fz)  "<F_R>"
  F/1(Fx) -> Bus Creator13/1
  R/1(Fx) -> Bus Creator13/2
  Bus Creator14/1 -> Fs/1
  F/2(Fy) -> Gain/1
  R/2(Fy) -> Gain1/1
  F/3(My) -> Bus Creator15/1
  R/3(My) -> Bus Creator15/2
  R/4(alpha) -> Bus Creator16/2
  R/5(r_dyn) -> Bus Creator17/2
  F/5(r_dyn) -> Bus Creator17/1
  Bus Creator15/1 -> My/1
  F/4(alpha) -> Bus Creator16/1
  Bus Creator16/1 -> alpha/1
  Bus Creator17/1 -> r_dyn/1
  Bus Creator19/1 -> r_stat/1
  F/6(r_stat) -> Bus Creator19/1
  R/6(r_stat) -> Bus Creator19/2
  Bus Creator13/1 -> Fl/1
  M_brems/1 -> Bus Selector11/1
  M_antr/1 -> Bus Selector12/1
  Bus Selector11/1 -> F/2(M_brems)  "<M_brems_F>"
  Bus Selector12/1 -> F/3(M_antr)  "<M_antr_F>"
  Bus Selector12/2 -> R/6(M_antr)  "<M_antr_R>"
  Bus Selector11/2 -> R/5(M_brems)  "<M_brems_R>"
  Bus Selector2/1 -> R/3(beta), F/5(beta)  "<SideSlipAngleBeta [rad]>"
  Bus Selector/1 -> R/2(psip), F/6(psip)  "<YawAngleVelocityPsip [rad/s]>"
  vabs/1 -> R/1(vabs), F/7(vabs)
  delta/1 -> F/4(delta)
  TIR_parameter/1 -> Bus Selector1/1
  Bus Selector1/1 -> F/8(TIR_parameter)  "<front>"
  Bus Selector1/2 -> R/7(TIR_parameter)  "<rear>"

== system Single_Track_Model_linear/SingleTrackModel_linear/vehicle_model/wheel/calc_omega ==
  vl : Inport
  r_dyn : Inport  Port=2
  Bus Creator : BusCreator  Inputs=2
  Bus Selector : BusSelector  OutputSignals=vl_F,vl_R
  Bus Selector6 : BusSelector  OutputSignals=r_dyn_F,r_dyn_R
  Divide1 : Product  Inputs=*/
  Divide3 : Product  Inputs=*/
  Unit Delay1 : UnitDelay  InitialCondition=0.3  SampleTime=-1
  Unit Delay3 : UnitDelay  InitialCondition=0.3  SampleTime=-1
  omega : Outport
  wires:
  Divide3/1 -> Bus Creator/2  "omega_R"
  Bus Selector/2 -> Divide3/1  "<vl_R>"
  Divide1/1 -> Bus Creator/1  "omega_F"
  Bus Selector/1 -> Divide1/1  "<vl_F>"
  vl/1 -> Bus Selector/1
  Bus Creator/1 -> omega/1
  Unit Delay1/1 -> Divide1/2
  Unit Delay3/1 -> Divide3/2
  r_dyn/1 -> Bus Selector6/1
  Bus Selector6/1 -> Unit Delay1/1  "<r_dyn_F>"
  Bus Selector6/2 -> Unit Delay3/1  "<r_dyn_R>"

== system Single_Track_Model_linear/SingleTrackModel_linear/vehicle_model/wheel/calc_v ==
  delta : Inport
  beta : Inport  Port=2
  psi : Inport  Port=3
  v : Inport  Port=4
  calc_vl : Subsystem
  calc_vs : Subsystem
  vl : Outport
  vs : Outport  Port=2
  wires:
  calc_vs/1(vs) -> vs/1
  beta/1 -> calc_vs/2(beta), calc_vl/4(beta)
  v/1 -> calc_vs/4(v), calc_vl/2(v)
  calc_vl/1(vl) -> vl/1
  [lR] -> calc_vs/6(lR)
  [lF] -> calc_vl/1(lF), calc_vs/5(lF)
  delta/1 -> calc_vs/1(delta), calc_vl/5(delta)
  psi/1 -> calc_vl/3(psi), calc_vs/3(psi)

== system Single_Track_Model_linear/SingleTrackModel_linear/vehicle_model/wheel/v0_korr ==
  vl : Inport
  omega : Inport  Port=2
  r_dyn : Inport  Port=3
  Bus Creator : BusCreator  Inputs=2
  Bus Selector : BusSelector  OutputSignals=vl_F,vl_R
  Bus Selector1 : BusSelector  OutputSignals=r_dyn_F,r_dyn_R
  Bus Selector2 : BusSelector  OutputSignals=omega_F,omega_R
  Subsystem2 : vehicle_model/vehicle_model/wheel/v0_korr/Subsystem4  SystemSampleTime=-1
  Subsystem4 : Subsystem
  v_low : Constant  Value=0.01  VectorParams1D=off
  omega_out : Outport
  wires:
  Subsystem2/1 -> Bus Creator/2  "omega_R [rad/s]"
  Subsystem4/1(omega_out) -> Bus Creator/1  "omega_F [rad/s]"
  Bus Selector2/2 -> Subsystem2/4  "<omega_R>"
  Bus Selector2/1 -> Subsystem4/4(omega)  "<omega_F>"
  Bus Selector1/2 -> Subsystem2/3  "<r_dyn_R>"
  Bus Selector1/1 -> Subsystem4/3(r_dyn)  "<r_dyn_F>"
  v_low/1 -> Subsystem2/2, Subsystem4/2(v_low)
  Bus Selector/2 -> Subsystem2/1  "<vl_R>"
  Bus Selector/1 -> Subsystem4/1(vl)  "<vl_F>"
  Bus Creator/1 -> omega_out/1
  omega/1 -> Bus Selector2/1
  r_dyn/1 -> Bus Selector1/1
  vl/1 -> Bus Selector/1

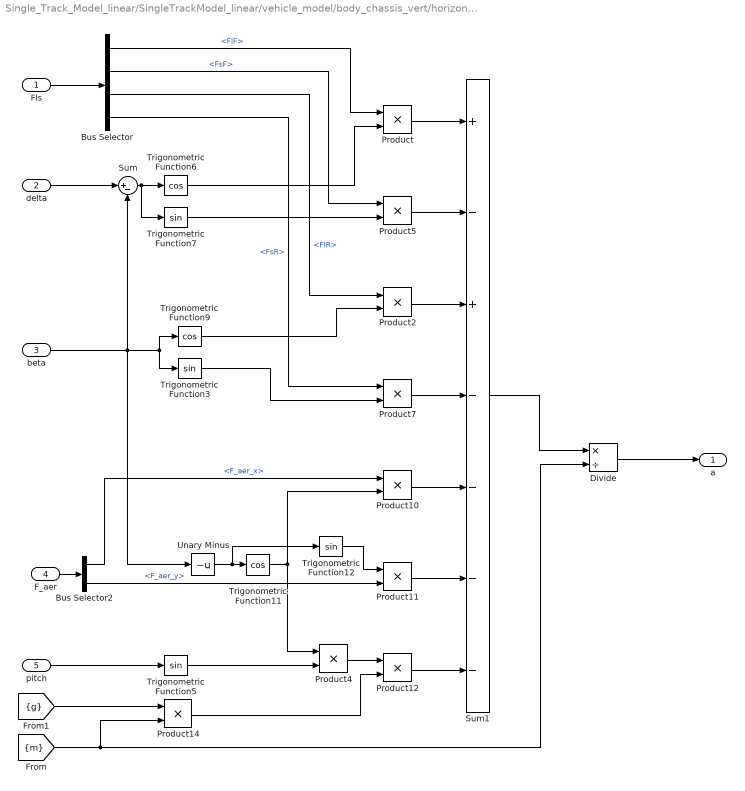
== system Single_Track_Model_linear/SingleTrackModel_linear/vehicle_model/body_chassis_vert/horizontal/acc ==
  Fls : Inport
  delta : Inport  Port=2
  beta : Inport  Port=3
  F_aer : Inport  Port=4
  pitch : Inport  Port=5
  Bus Selector : BusSelector  OutputSignals=Fl.FlF,Fs.FsF,Fl.FlR,Fs.FsR
  Bus Selector2 : BusSelector  OutputSignals=F_aer_x,F_aer_y
  Divide : Product  Inputs=*/
  Product{,2,4..5,7,10..12,14} (9 alike) : Product  RndMeth=Zero
  Sum : Sum  Inputs=|+-
  Sum1 : Sum  Inputs=+-+----
  Trigonometric Function11 : Trigonometry  Operator=cos
  Trigonometric Function{3,5,7,12} (4 alike) : Trigonometry
  Trigonometric Function6 : Trigonometry  Operator=cos
  Trigonometric Function9 : Trigonometry  Operator=cos
  Unary Minus : UnaryMinus
  a : Outport
  wires:
  Divide/1 -> a/1
  pitch/1 -> Trigonometric Function5/1
  [g] -> Product14/1
  Product14/1 -> Product12/2
  Product12/1 -> Sum1/7
  Product4/1 -> Product12/1
  Trigonometric Function5/1 -> Product4/2
  F_aer/1 -> Bus Selector2/1
  Unary Minus/1 -> Trigonometric Function11/1, Trigonometric Function12/1
  Trigonometric Function12/1 -> Product11/1
  Trigonometric Function11/1 -> Product10/2, Product4/1
  Bus Selector2/2 -> Product11/2  "<F_aer_y>"
  Bus Selector2/1 -> Product10/1  "<F_aer_x>"
  Product11/1 -> Sum1/6
  Trigonometric Function3/1 -> Product7/2
  beta/1 -> Unary Minus/1, Sum/2, Trigonometric Function3/1, Trigonometric Function9/1
  Sum1/1 -> Divide/1
  Product10/1 -> Sum1/5
  Product7/1 -> Sum1/4
  Trigonometric Function9/1 -> Product2/2
  Product2/1 -> Sum1/3
  Product5/1 -> Sum1/2
  Product/1 -> Sum1/1
  Trigonometric Function7/1 -> Product5/2
  Trigonometric Function6/1 -> Product/2
  Sum/1 -> Trigonometric Function7/1, Trigonometric Function6/1
  Fls/1 -> Bus Selector/1
  Bus Selector/1 -> Product/1  "<FlF>"
  Bus Selector/2 -> Product5/1  "<FsF>"
  Bus Selector/3 -> Product2/1  "<FlR>"
  Bus Selector/4 -> Product7/1  "<FsR>"
  delta/1 -> Sum/1
  [m] -> Product14/2, Divide/2

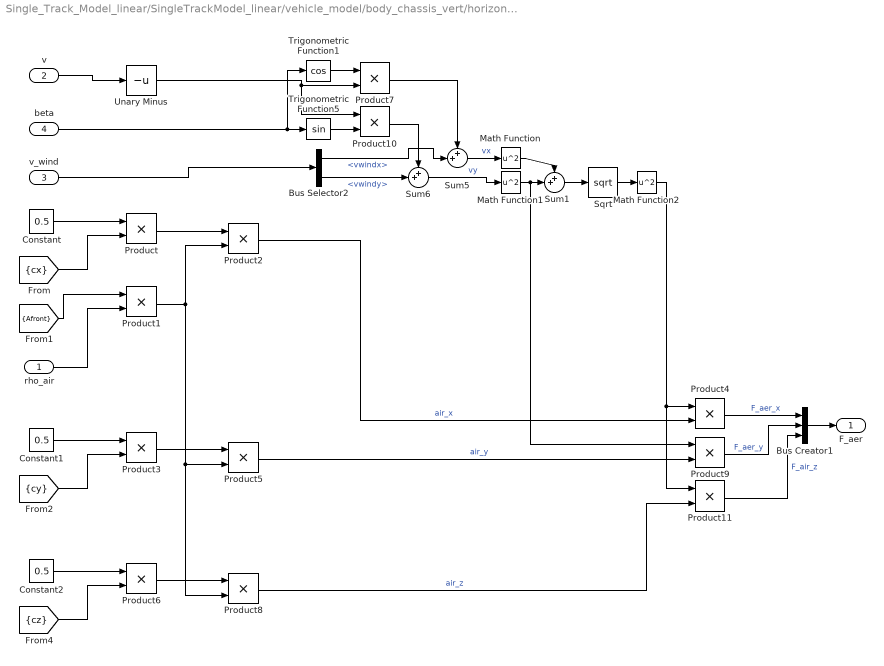
== system Single_Track_Model_linear/SingleTrackModel_linear/vehicle_model/body_chassis_vert/horizontal/aerodynamics ==
  rho_air : Inport
  v : Inport  Port=2
  v_wind : Inport  Port=3
  beta : Inport  Port=4
  Bus Creator1 : BusCreator  Inputs=3
  Bus Selector2 : BusSelector  OutputSignals=vwindx,vwindy
  Constant : Constant  Value=0.5
  Constant1 : Constant  Value=0.5
  Constant2 : Constant  Value=0.5
  Math Function : Math  Operator=square  SaturateOnIntegerOverflow=on
  Math Function1 : Math  Operator=square  SaturateOnIntegerOverflow=on
  Math Function2 : Math  Operator=square  SaturateOnIntegerOverflow=on
  Product{,1..11} (12 alike) : Product  RndMeth=Zero
  Sqrt : Sqrt  SaturateOnIntegerOverflow=on
  Sum1 : Sum  Inputs=++|
  Sum5 : Sum  Inputs=++|
  Sum6 : Sum  Inputs=++|
  Trigonometric Function1 : Trigonometry  Operator=cos
  Trigonometric Function5 : Trigonometry
  Unary Minus : UnaryMinus
  F_aer : Outport
  wires:
  Unary Minus/1 -> Product10/1, Product7/2
  Product11/1 -> Bus Creator1/3  "F_air_z"
  Math Function2/1 -> Product11/1, Product4/1
  Sqrt/1 -> Math Function2/1
  Sum1/1 -> Sqrt/1
  Math Function/1 -> Sum1/1
  Math Function1/1 -> Product9/1, Sum1/2
  Product7/1 -> Sum5/1
  Product10/1 -> Sum6/1
  v/1 -> Unary Minus/1
  Trigonometric Function1/1 -> Product7/1
  Trigonometric Function5/1 -> Product10/2
  Bus Creator1/1 -> F_aer/1
  Product9/1 -> Bus Creator1/2  "F_aer_y"
  Product4/1 -> Bus Creator1/1  "F_aer_x"
  Sum6/1 -> Math Function1/1  "vy"
  Sum5/1 -> Math Function/1  "vx"
  Bus Selector2/1 -> Sum5/2  "<vwindx>"
  Bus Selector2/2 -> Sum6/2  "<vwindy>"
  beta/1 -> Trigonometric Function1/1, Trigonometric Function5/1
  v_wind/1 -> Bus Selector2/1
  Product8/1 -> Product11/2  "air_z"
  Product6/1 -> Product8/1
  [cz] -> Product6/2
  Constant2/1 -> Product6/1
  Product5/1 -> Product9/2  "air_y"
  Product3/1 -> Product5/1
  [cy] -> Product3/2
  Constant1/1 -> Product3/1
  Product2/1 -> Product4/2  "air_x"
  Product1/1 -> Product8/2, Product5/2, Product2/2
  Product/1 -> Product2/1
  rho_air/1 -> Product1/2
  [Afront] -> Product1/1
  [cx] -> Product/2
  Constant/1 -> Product/1

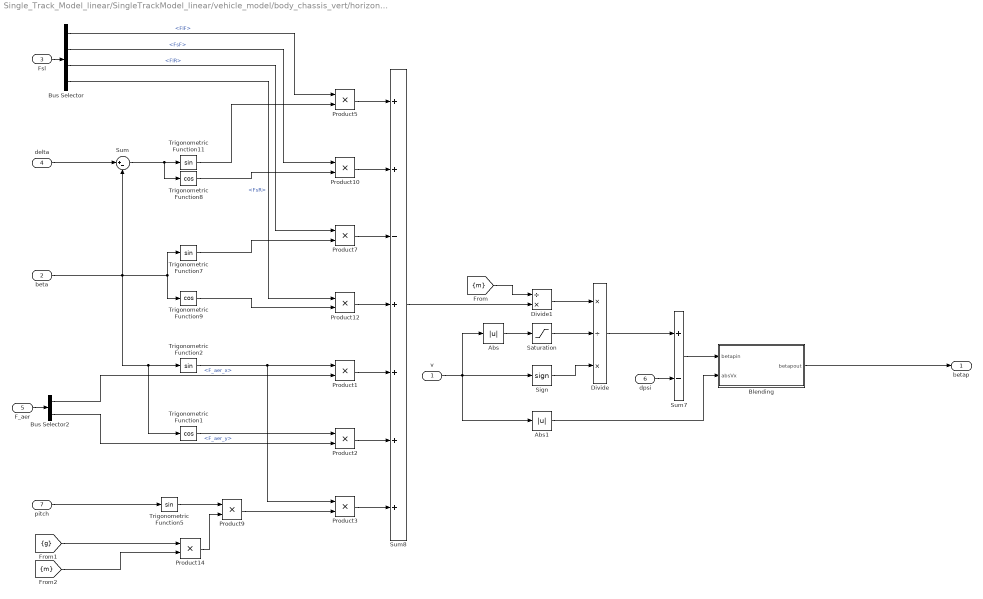
== system Single_Track_Model_linear/SingleTrackModel_linear/vehicle_model/body_chassis_vert/horizontal/betap ==
  v : Inport
  beta : Inport  Port=2
  Fsl : Inport  Port=3
  delta : Inport  Port=4
  F_aer : Inport  Port=5
  dpsi : Inport  Port=6
  pitch : Inport  Port=7
  Abs : Abs
  Abs1 : Abs
  Blending : Subsystem
  Bus Selector : BusSelector  OutputSignals=Fl.FlF,Fs.FsF,Fl.FlR,Fs.FsR
  Bus Selector2 : BusSelector  OutputSignals=F_aer_x,F_aer_y
  Divide : Product  Inputs=*/*
  Divide1 : Product  Inputs=/*
  Product{1..3,5,7,9..10,12,14} (9 alike) : Product  RndMeth=Zero
  Saturation : Saturate  UpperLimit=1e10  LowerLimit=0.5e-5
  Sign : Signum
  Sum : Sum  Inputs=|+-
  Sum7 : Sum  Inputs=+-
  Sum8 : Sum  Inputs=++-++++
  Trigonometric Function1 : Trigonometry  Operator=cos
  Trigonometric Function{2,5,7,11} (4 alike) : Trigonometry
  Trigonometric Function8 : Trigonometry  Operator=cos
  Trigonometric Function9 : Trigonometry  Operator=cos
  betap : Outport
  wires:
  Blending/1(betapout) -> betap/1
  pitch/1 -> Trigonometric Function5/1
  Product14/1 -> Product9/2
  Product9/1 -> Product3/2
  Trigonometric Function5/1 -> Product9/1
  [g] -> Product14/1
  [m] -> Product14/2
  Product3/1 -> Sum8/7
  Sign/1 -> Divide/3
  Sum7/1 -> Blending/1(betapin)
  Abs1/1 -> Blending/2(absVx)
  Abs/1 -> Saturation/1
  Trigonometric Function1/1 -> Product2/1
  Bus Selector2/2 -> Product2/2  "<F_aer_y>"
  Trigonometric Function2/1 -> Product3/1, Product1/1
  Bus Selector2/1 -> Product1/2  "<F_aer_x>"
  Product2/1 -> Sum8/6
  F_aer/1 -> Bus Selector2/1
  v/1 -> Abs/1, Abs1/1, Sign/1
  Saturation/1 -> Divide/2
  Divide/1 -> Sum7/1
  dpsi/1 -> Sum7/2
  Trigonometric Function9/1 -> Product12/2
  beta/1 -> Trigonometric Function1/1, Trigonometric Function2/1, Sum/2, Trigonometric Function7/1, Trigonometric Function9/1
  Sum8/1 -> Divide1/2
  Product1/1 -> Sum8/5
  Product12/1 -> Sum8/4
  Trigonometric Function7/1 -> Product7/2
  Product7/1 -> Sum8/3
  Product10/1 -> Sum8/2
  Product5/1 -> Sum8/1
  Trigonometric Function8/1 -> Product10/2
  Trigonometric Function11/1 -> Product5/2
  Sum/1 -> Trigonometric Function11/1, Trigonometric Function8/1
  Divide1/1 -> Divide/1
  delta/1 -> Sum/1
  Fsl/1 -> Bus Selector/1
  Bus Selector/1 -> Product5/1  "<FlF>"
  Bus Selector/2 -> Product10/1  "<FsF>"
  Bus Selector/3 -> Product7/1  "<FlR>"
  Bus Selector/4 -> Product12/1  "<FsR>"
  [m] -> Divide1/1
